simulink model "aconserversimulation"  (R2019b)
settings: Solver=FixedStepAuto  StartTime=0.0  StopTime=30  RelTol=1e-3
undefined symbols (not defined in the file or in its folder): Acid, Lead, sigbuilder_block
libraries: powerlib x39, simulink x14, powerlib_extras x9, electricdrivelib x3, re_lib x1
(part 2 of 2)

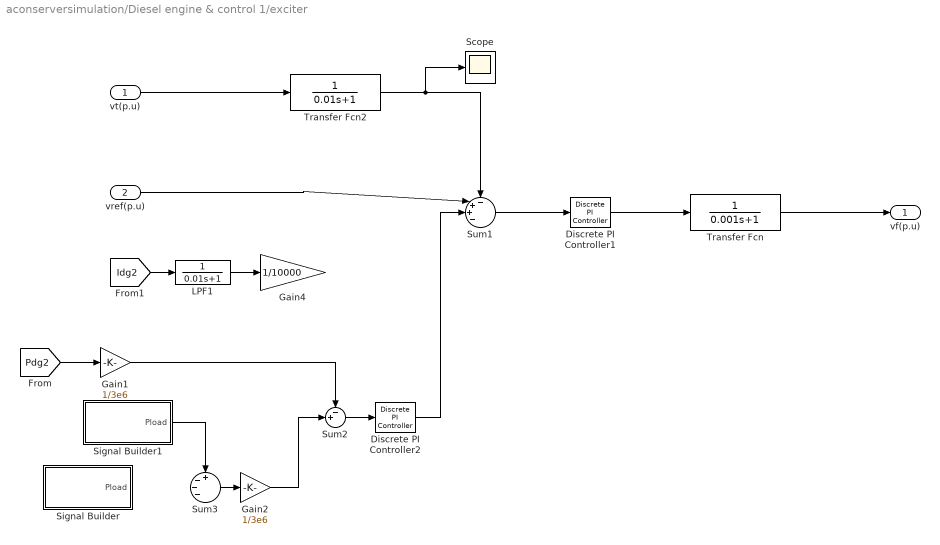
== system aconserversimulation/Diesel engine & control 1/exciter ==
  vt(p.u) : Inport
  vref(p.u) : Inport  Port=2
  Discrete PI Controller1 : powerlib_extras/Discrete  Control Blocks/Discrete PI Controller  Kp=30  Ki=10  Par_Limits=[10 -10]  Init=0  Ts=5e-6
      settings: SourceProductName=Simscape Electrical
  Discrete PI Controller2 : powerlib_extras/Discrete  Control Blocks/Discrete PI Controller  Kp=30  Ki=10  Par_Limits=[10 -10]  Init=0  Ts=5e-6
      settings: SourceProductName=Simscape Electrical
  Gain1 : Gain  Gain=1/3e6
  Gain2 : Gain  Gain=1/3e6
  Gain4 : Gain  Gain=1/10000
  LPF1 : TransferFcn  Denominator=[0.01 1]
  Scope : Scope
  Signal Builder : Subsystem  Tag=STV Subsys  LoadFcn=sigbuilder_block('load');  StartFcn=sigbuilder_block('start');  StopFcn=sigbuilder_block('stop');  ClipboardFcn=sigbuilder_block('clipboard');  mask(Sigbuilder block){tuvar=[0:10]}
      mask help: Simulink:masks:SigbuilderBlock_MD
      mask init:
      | if ~strcmp(get_param(bdroot(gcbh),'SimulationStatus'),'stopped') tuvar = sigbuilder_block('maskInit'); end
      settings: CopyFcn=sigbuilder_block('copy');  DeleteFcn=sigbuilder_block('delete');  ModelCloseFcn=sigbuilder_block('modelClose');  PreSaveFcn=sigbuilder_block('preSave');  PauseFcn=sigbuilder_block('pause');  ContinueFcn=sigbuilder_block('continue');  NameChangeFcn=sigbuilder_block('namechange');  OpenFcn=sigbuilder_block('open',[381.6 135 550.8 400.2 ]);  CloseFcn=sigbuilder_block('close');
      mask Display: plot(0, 0, 100, 100,[2, 2, 32, 32, 2], [68, 8, 8, 68, 68],[32, 2], [38, 38], [32, 19, 2],[53, 60, 44], [32, 17, 17, 2],[16, 16, 31, 31]);txt = getActiveGroup(gcbh);text(2, 100, txt,'verticalAlignment', 'top');
  Signal Builder1 : Subsystem  Tag=STV Subsys  LoadFcn=sigbuilder_block('load');  StartFcn=sigbuilder_block('start');  StopFcn=sigbuilder_block('stop');  ClipboardFcn=sigbuilder_block('clipboard');  mask(Sigbuilder block){tuvar=[0:10]}
      mask help: Simulink:masks:SigbuilderBlock_MD
      mask init:
      | if ~strcmp(get_param(bdroot(gcbh),'SimulationStatus'),'stopped') tuvar = sigbuilder_block('maskInit'); end
      settings: CopyFcn=sigbuilder_block('copy');  DeleteFcn=sigbuilder_block('delete');  ModelCloseFcn=sigbuilder_block('modelClose');  PreSaveFcn=sigbuilder_block('preSave');  PauseFcn=sigbuilder_block('pause');  ContinueFcn=sigbuilder_block('continue');  NameChangeFcn=sigbuilder_block('namechange');  OpenFcn=sigbuilder_block('open',[381.6 135 550.8 400.2 ]);  CloseFcn=sigbuilder_block('close');
      mask Display: plot(0, 0, 100, 100,[2, 2, 32, 32, 2], [68, 8, 8, 68, 68],[32, 2], [38, 38], [32, 19, 2],[53, 60, 44], [32, 17, 17, 2],[16, 16, 31, 31]);txt = getActiveGroup(gcbh);text(2, 100, txt,'verticalAlignment', 'top');
  Sum1 : Sum  Inputs=-++-|
  Sum2 : Sum  Inputs=-+|
  Sum3 : Sum  Inputs=+---|
  Transfer Fcn : TransferFcn  Denominator=[0.001 1]
  Transfer Fcn2 : TransferFcn  Denominator=[0.01 1]
  vf(p.u) : Outport  VectorParamsAs1DForOutWhenUnconnected=off
  wires:
  vt(p.u)/1 -> Transfer Fcn2/1
  Sum1/1 -> Discrete PI Controller1/1
  Discrete PI Controller1/1 -> Transfer Fcn/1
  Transfer Fcn/1 -> vf(p.u)/1
  vref(p.u)/1 -> Sum1/2
  Transfer Fcn2/1 -> Scope/1, Sum1/1
  Sum2/1 -> Discrete PI Controller2/1
  [Pdg2] -> Gain1/1
  Gain1/1 -> Sum2/1
  [Idg2] -> LPF1/1
  LPF1/1 -> Gain4/1
  Discrete PI Controller2/1 -> Sum1/3
  Sum3/1 -> Gain2/1
  Gain2/1 -> Sum2/2
  Signal Builder1/1(Pload) -> Sum3/1

== system aconserversimulation/SC2/Buck-Boost 1  ==
  Vbus_ref : Inport
  Vbus_mes : Inport  Port=2
  Buck-Boost : Subsystem
  Current Measurement : powerlib/Measurements/Current Measurement  PhasorSimulation=off  OutputType=Complex  PSBequivalent=0
      settings: SourceProductName=Simscape Electrical
  Current loop : Subsystem
  Scope3 : Scope
  Voltage loop : Subsystem
  Vout+ : PMIOPort  Side=Right
  Vin+ : PMIOPort  Port=2  Side=Left
  Vout- : PMIOPort  Port=3  Side=Right
  Vin- : PMIOPort  Port=4  Side=Left
  wires:
  Current Measurement/1 -> Current loop/2(iLmes)
  Vbus_mes/1 -> Voltage loop/2(Vmes)
  Vbus_ref/1 -> Voltage loop/1(Vref)
  Current loop/1(d) -> Buck-Boost/1(d)
  Voltage loop/1(iLref) -> Scope3/1, Current loop/1(iLref)
  connections:
  Buck-Boost/RConn1 -- Vout+/RConn1
  Buck-Boost/RConn2 -- Vout-/RConn1
  Vin-/RConn1 -- Buck-Boost/LConn2
  Current Measurement/RConn1 -- Buck-Boost/LConn1
  Current Measurement/LConn1 -- Vin+/RConn1

== system aconserversimulation/Subsystem/Signal Builder ==
  Demux : Demux  Tag=STV Demux  Outputs=1
  FromWs : FromWorkspace  Tag=STV FromWs  VariableName=tuvar  SampleTime=0
      SigBuilderData=|
      | common.afterFinalStr = 'Extrapolate'
      | common.sampleTime = 0
      | dataSet.timeRange = [0 30]
      | dataSet.name = 'Group 1'
      | sbobj.Groups.Name = 'Group 1'
      | sbobj.Groups.Signals.Name = 'Pload'
      | sbobj.Groups.Signals.XData = [0 10 14 16 18.75 21 21 26 26 30]
      | sbobj.Groups.Signals.YData = [0 0 3000000 3000000 6000000 6000000 2000000 2000000 6000000 6020000]
      | sbobj.Groups.TimeRange = [0 30]
  Pload : Outport  Tag=STV Outport  VectorParamsAs1DForOutWhenUnconnected=off
  wires:
  Demux/1 -> Pload/1
  FromWs/1 -> Demux/1

== system aconserversimulation/Battery_V/Buck-Boost 2/Buck-Boost ==
  d : Inport
  Add2 : Sum  Inputs=+-
  Constant : Constant
  Mosfet1 : powerlib/Power Electronics/Mosfet  Ron=0.1  Lon=0  Rd=0.01  Vfd=0  IC=0  Rs=1e5  Cs=inf  Measurements=on
      settings: SourceProductName=Simscape Electrical
  Mosfet3 : powerlib/Power Electronics/Mosfet  Ron=0.1  Lon=0  Rd=0.01  Vfd=0  IC=0  Rs=1e5  Cs=inf  Measurements=on
      settings: SourceProductName=Simscape Electrical
  Relational Operator : RelationalOperator  OutDataTypeStr=boolean  RndMeth=Nearest
  Repeating Sequence : simulink/Sources/Repeating Sequence  rep_seq_t=[0 0.0005 0.001]  rep_seq_y=[0 1 0]
  Terminator : Terminator
  Terminator1 : Terminator
  Vout+ : PMIOPort  Side=Right
  Vout- : PMIOPort  Port=2  Side=Right
  Vin+ : PMIOPort  Port=3  Side=Left
  Vin- : PMIOPort  Port=4  Side=Left
  wires:
  Relational Operator/1 -> Mosfet1/1, Add2/2
  Repeating Sequence/1 -> Relational Operator/2
  Constant/1 -> Add2/1
  Add2/1 -> Mosfet3/1
  Mosfet1/1 -> Terminator1/1
  Mosfet3/1 -> Terminator/1
  d/1 -> Relational Operator/1
  connections:
  Mosfet1/RConn1 -- Vin-/RConn1 -- Vout-/RConn1
  Mosfet3/RConn1 -- Vin+/RConn1 -- Mosfet1/LConn1
  Vout+/RConn1 -- Mosfet3/LConn1

== system aconserversimulation/Battery_V/Buck-Boost 2/Current loop ==
  note: 原p/i=0.0015/0.2
  Iref : Inport
  imes : Inport  Port=2
  Add1 : Sum  Inputs=+-
  Discrete PID Controller1 : simulink/Continuous/PID Controller  Controller=PI  Form=Parallel  TimeDomain=Continuous-time  SampleTime=-1  IntegratorMethod=Forward Euler  FilterMethod=Forward Euler  ControllerParametersSource=internal  P=1.5  I=1  D=0  UseFilter=on  N=100  TunerSelectOption=Transfer Function Based (PID Tuner App)  InitialConditionSource=internal  InitialConditionForIntegrator=0  InitialConditionForFilter=0  DifferentiatorICPrevScaledInput=0  ExternalReset=none  TrackingMode=off  Kt=1  LimitOutput=off  UpperSaturationLimit=inf  LowerSaturationLimit=-inf  LinearizeAsGain=off  AntiWindupMode=none  Kb=1  POutMin=[]  POutMax=[]  IOutMin=[]  IOutMax=[]  DOutMin=[]  DOutMax=[]  NOutMin=[]  NOutMax=[]  SumOutMin=[]  SumOutMax=[]  SaturationOutMin=[]  SaturationOutMax=[]  PParamMin=[]  PParamMax=[]  IParamMin=[]  IParamMax=[]  DParamMin=[]  DParamMax=[]  NParamMin=[]  NParamMax=[]  KbParamMin=[]  KbParamMax=[]  KtParamMin=[]  KtParamMax=[]  KbOutMin=[]  KbOutMax=[]  KtOutMin=[]  KtOutMax=[]  IntegratorOutMin=[]  IntegratorOutMax=[]  FilterOutMin=[]  FilterOutMax=[]  SumI1OutMin=[]  SumI1OutMax=[]  SumI2OutMin=[]  SumI2OutMax=[]  SumI3OutMin=[]  SumI3OutMax=[]  SumI4OutMin=[]  SumI4OutMax=[]  SumDOutMin=[]  SumDOutMax=[]  DifferentiatorOutMin=[]  DifferentiatorOutMax=[]  FilterDiffOutCoefMin=[]  FilterDiffOutCoefMax=[]  ReciprocalOutMin=[]  ReciprocalOutMax=[]  SumDenOutMin=[]  SumDenOutMax=[]  SumNumOutMin=[]  SumNumOutMax=[]  DivideOutMin=[]  DivideOutMax=[]  IntegratorContinuousStateAttributes=''  IntegratorStateMustResolveToSignalObject=off  IntegratorRTWStateStorageClass=Auto  FilterContinuousStateAttributes=''  FilterStateMustResolveToSignalObject=off  FilterRTWStateStorageClass=Auto  ParallelPVariant=InternalParameters  IdealPVariant=Disabled  IVariant=InternalParameters  DVariant=Disabled  IntegratorVariant=Continuous  SatVariant=Disabled  AWVariant=Passthrough  PCopyVariant=Disabled  TRVariant=Disabled  FdbkBlocksVariant=Forward  IdealPFdbkVariant=Disabled  SatFdbkVariant=Disabled  DerivativeFilterVariant=Disabled  NVariant=Disabled  NCopyVariant=Disabled_SignalSpec  FilterICVariant=Disabled  IntegratorICVariant=InternalICs  ExternalResetVariant=Disabled  TRSumVariant=Passthrough  SumFdbkVariant=Disabled  SumVariant=Sum_PI
  d : Outport  VectorParamsAs1DForOutWhenUnconnected=off
  wires:
  Discrete PID Controller1/1 -> d/1
  imes/1 -> Add1/2
  Add1/1 -> Discrete PID Controller1/1
  Iref/1 -> Add1/1

== system aconserversimulation/Battery_V/Buck-Boost 2/Current loop1 ==
  note: 原p/i=0.0015/0.2
  Iref : Inport
  imes : Inport  Port=2
  Add1 : Sum  Inputs=+-
  Discrete PID Controller1 : simulink/Continuous/PID Controller  Controller=PI  TimeDomain=Continuous-time  SampleTime=-1  IntegratorMethod=Forward Euler  FilterMethod=Forward Euler  Form=Parallel  UseFilter=on  ControllerParametersSource=internal  P=100  I=10  D=0  N=100  InitialConditionSource=internal  InitialConditionForIntegrator=0  InitialConditionForFilter=0  ExternalReset=none  LimitOutput=off  UpperSaturationLimit=inf  LowerSaturationLimit=-inf  LinearizeAsGain=off  AntiWindupMode=none  Kb=1  TrackingMode=off  Kt=1  PParamMin=[]  PParamMax=[]  IParamMin=[]  IParamMax=[]  DParamMin=[]  DParamMax=[]  NParamMin=[]  NParamMax=[]  KbParamMin=[]  KbParamMax=[]  KtParamMin=[]  KtParamMax=[]  POutMin=[]  POutMax=[]  IOutMin=[]  IOutMax=[]  DOutMin=[]  DOutMax=[]  NOutMin=[]  NOutMax=[]  KbOutMin=[]  KbOutMax=[]  KtOutMin=[]  KtOutMax=[]  IntegratorOutMin=[]  IntegratorOutMax=[]  FilterOutMin=[]  FilterOutMax=[]  SumOutMin=[]  SumOutMax=[]  SumI1OutMin=[]  SumI1OutMax=[]  SumI2OutMin=[]  SumI2OutMax=[]  SumI3OutMin=[]  SumI3OutMax=[]  SumDOutMin=[]  SumDOutMax=[]  SaturationOutMin=[]  SaturationOutMax=[]  IntegratorContinuousStateAttributes=''  IntegratorStateMustResolveToSignalObject=off  IntegratorRTWStateStorageClass=Auto  FilterContinuousStateAttributes=''  FilterStateMustResolveToSignalObject=off  FilterRTWStateStorageClass=Auto  DifferentiatorICPrevScaledInput=0  DifferentiatorOutMin=[]  DifferentiatorOutMax=[]  InitialConditionSetting=State (most efficient)  FilterDiffOutCoefMin=[]  FilterDiffOutCoefMax=[]  SumDenOutMin=[]  SumDenOutMax=[]  SumNumOutMin=[]  SumNumOutMax=[]  ReciprocalOutMin=[]  ReciprocalOutMax=[]  DivideOutMin=[]  DivideOutMax=[]  TunerSelectOption=Transfer Function Based (PID Tuner App)
  Saturation : Saturate  UpperLimit=500  LowerLimit=-500
  Scope : Scope
  d : Outport  VectorParamsAs1DForOutWhenUnconnected=off
  wires:
  Discrete PID Controller1/1 -> Saturation/1
  imes/1 -> Add1/2
  Add1/1 -> Discrete PID Controller1/1
  Iref/1 -> Add1/1
  [P] -> Scope/1
  Saturation/1 -> d/1

== system aconserversimulation/Battery_V/Buck-Boost 2/Voltage loop ==
  Vref : Inport
  Vmes : Inport  Port=2
  Add : Sum  Inputs=+-
  Discrete PI Controller : powerlib_extras/Discrete  Control Blocks/Discrete PI Controller  Kp=10  Ki=10  Par_Limits=[500 -500]  Init=0  Ts=5e-6
      settings: SourceProductName=Simscape Electrical
  Discrete PID Controller1 : simulink/Continuous/PID Controller  Controller=PI  Form=Parallel  TimeDomain=Continuous-time  SampleTime=-1  IntegratorMethod=Forward Euler  FilterMethod=Forward Euler  ControllerParametersSource=internal  P=10  I=10  D=0  UseFilter=on  N=100  TunerSelectOption=Transfer Function Based (PID Tuner App)  InitialConditionSource=internal  InitialConditionForIntegrator=0  InitialConditionForFilter=0  DifferentiatorICPrevScaledInput=0  ExternalReset=none  TrackingMode=off  Kt=1  LimitOutput=off  UpperSaturationLimit=inf  LowerSaturationLimit=-inf  LinearizeAsGain=off  AntiWindupMode=none  Kb=1  POutMin=[]  POutMax=[]  IOutMin=[]  IOutMax=[]  DOutMin=[]  DOutMax=[]  NOutMin=[]  NOutMax=[]  SumOutMin=[]  SumOutMax=[]  SaturationOutMin=[]  SaturationOutMax=[]  PParamMin=[]  PParamMax=[]  IParamMin=[]  IParamMax=[]  DParamMin=[]  DParamMax=[]  NParamMin=[]  NParamMax=[]  KbParamMin=[]  KbParamMax=[]  KtParamMin=[]  KtParamMax=[]  KbOutMin=[]  KbOutMax=[]  KtOutMin=[]  KtOutMax=[]  IntegratorOutMin=[]  IntegratorOutMax=[]  FilterOutMin=[]  FilterOutMax=[]  SumI1OutMin=[]  SumI1OutMax=[]  SumI2OutMin=[]  SumI2OutMax=[]  SumI3OutMin=[]  SumI3OutMax=[]  SumI4OutMin=[]  SumI4OutMax=[]  SumDOutMin=[]  SumDOutMax=[]  DifferentiatorOutMin=[]  DifferentiatorOutMax=[]  FilterDiffOutCoefMin=[]  FilterDiffOutCoefMax=[]  ReciprocalOutMin=[]  ReciprocalOutMax=[]  SumDenOutMin=[]  SumDenOutMax=[]  SumNumOutMin=[]  SumNumOutMax=[]  DivideOutMin=[]  DivideOutMax=[]  IntegratorContinuousStateAttributes=''  IntegratorStateMustResolveToSignalObject=off  IntegratorRTWStateStorageClass=Auto  FilterContinuousStateAttributes=''  FilterStateMustResolveToSignalObject=off  FilterRTWStateStorageClass=Auto  ParallelPVariant=InternalParameters  IdealPVariant=Disabled  IVariant=InternalParameters  DVariant=Disabled  IntegratorVariant=Continuous  SatVariant=Disabled  AWVariant=Passthrough  PCopyVariant=Disabled  TRVariant=Disabled  FdbkBlocksVariant=Forward  IdealPFdbkVariant=Disabled  SatFdbkVariant=Disabled  DerivativeFilterVariant=Disabled  NVariant=Disabled  NCopyVariant=Disabled_SignalSpec  FilterICVariant=Disabled  IntegratorICVariant=InternalICs  ExternalResetVariant=Disabled  TRSumVariant=Passthrough  SumFdbkVariant=Disabled  SumVariant=Sum_PI
  HPF2 : TransferFcn  Denominator=[2 1]
  Iref : Outport  VectorParamsAs1DForOutWhenUnconnected=off
  wires:
  Vref/1 -> Add/1
  Vmes/1 -> Add/2
  Discrete PI Controller/1 -> Iref/1
  Add/1 -> HPF2/1
  HPF2/1 -> Discrete PI Controller/1

== system aconserversimulation/Diesel engine & control /exciter/Signal Builder ==
  Demux : Demux  Tag=STV Demux  Outputs=1
  FromWs : FromWorkspace  Tag=STV FromWs  VariableName=tuvar  SampleTime=0
      SigBuilderData=|
      | common.afterFinalStr = 'Extrapolate'
      | common.sampleTime = 0
      | dataSet.timeRange = [0 20]
      | dataSet.name = 'Group 1'
      | sbobj.Groups.Name = 'Group 1'
      | sbobj.Groups.Signals.Name = 'Pload'
      | sbobj.Groups.Signals.XData = [0 4 6 6.45 12 12 16 16 20]
      | sbobj.Groups.Signals.YData = [0.195 3000000 3000000 3000000 3000000 1500000 1500000 3000000 3000000]
      | sbobj.Groups.TimeRange = [0 20]
  Pload : Outport  Tag=STV Outport  VectorParamsAs1DForOutWhenUnconnected=off
  wires:
  Demux/1 -> Pload/1
  FromWs/1 -> Demux/1

== system aconserversimulation/Diesel engine & control /exciter/Signal Builder1 ==
  Demux : Demux  Tag=STV Demux  Outputs=1
  FromWs : FromWorkspace  Tag=STV FromWs  VariableName=tuvar  SampleTime=0
      SigBuilderData=|
      | common.afterFinalStr = 'Extrapolate'
      | common.sampleTime = 0
      | dataSet.timeRange = [0 30]
      | dataSet.name = 'Group 1'
      | sbobj.Groups.Name = 'Group 1'
      | sbobj.Groups.Signals.Name = 'Pload'
      | sbobj.Groups.Signals.XData = [0 10 14 16 16.45 22 22 26 26 30]
      | sbobj.Groups.Signals.YData = [0 0 2500000 2500000 3000000 3000000 1500000 1500000 3000000 3000000]
      | sbobj.Groups.TimeRange = [0 30]
  Pload : Outport  Tag=STV Outport  VectorParamsAs1DForOutWhenUnconnected=off
  wires:
  Demux/1 -> Pload/1
  FromWs/1 -> Demux/1

== system aconserversimulation/Diesel engine & control 1/exciter/Signal Builder ==
  Demux : Demux  Tag=STV Demux  Outputs=1
  FromWs : FromWorkspace  Tag=STV FromWs  VariableName=tuvar  SampleTime=0
      SigBuilderData=|
      | common.afterFinalStr = 'Extrapolate'
      | common.sampleTime = 0
      | dataSet.timeRange = [0 20]
      | dataSet.name = 'Group 1'
      | sbobj.Groups.Name = 'Group 1'
      | sbobj.Groups.Signals.Name = 'Pload'
      | sbobj.Groups.Signals.XData = [0 4 6 8.75 12 12 16 16 20]
      | sbobj.Groups.Signals.YData = [0.195 0 0 2500000 2500000 0 0 2500000 2500000]
      | sbobj.Groups.TimeRange = [0 20]
  Pload : Outport  Tag=STV Outport  VectorParamsAs1DForOutWhenUnconnected=off
  wires:
  Demux/1 -> Pload/1
  FromWs/1 -> Demux/1

== system aconserversimulation/Diesel engine & control 1/exciter/Signal Builder1 ==
  Demux : Demux  Tag=STV Demux  Outputs=1
  FromWs : FromWorkspace  Tag=STV FromWs  VariableName=tuvar  SampleTime=0
      SigBuilderData=|
      | common.afterFinalStr = 'Extrapolate'
      | common.sampleTime = 0
      | dataSet.timeRange = [0 30]
      | dataSet.name = 'Group 1'
      | sbobj.Groups.Name = 'Group 1'
      | sbobj.Groups.Signals.Name = 'Pload'
      | sbobj.Groups.Signals.XData = [0 4 16 18.75 22 22 26 26 30]
      | sbobj.Groups.Signals.YData = [0.195 0 0 2500000 2500000 0 0 2500000 2500000]
      | sbobj.Groups.TimeRange = [0 30]
  Pload : Outport  Tag=STV Outport  VectorParamsAs1DForOutWhenUnconnected=off
  wires:
  Demux/1 -> Pload/1
  FromWs/1 -> Demux/1

== system aconserversimulation/SC2/Buck-Boost 1 /Buck-Boost ==
  note: d
  note: 1-d
  d : Inport
  Constant : Constant
  L : powerlib/Elements/Series RLC Branch  LConnTagsString=__new0  RConnTagsString=__new0  BranchType=L  Resistance=1  Inductance=9e-3  SetiL0=off  InitialCurrent=0  Capacitance=1e-6  Setx0=off  InitialVoltage=0  Measurements=Branch current
      settings: SourceProductName=Simscape Electrical
  Mosfet : powerlib/Power Electronics/Mosfet  Ron=0.0001  Lon=0  Rd=0.0001  Vfd=0  IC=0  Rs=1e5  Cs=inf  Measurements=on
      settings: SourceProductName=Simscape Electrical
  Mosfet1 : powerlib/Power Electronics/Mosfet  Ron=0.0001  Lon=0  Rd=0.0001  Vfd=0  IC=0  Rs=1e5  Cs=inf  Measurements=on
      settings: SourceProductName=Simscape Electrical
  Relational Operator1 : RelationalOperator  OutDataTypeStr=boolean  RndMeth=Nearest
  Repeating Sequence1 : simulink/Sources/Repeating Sequence  rep_seq_t=[0 5e-4 1e-3]  rep_seq_y=[0 1 0]
  Sum : Sum  Inputs=|-+
  Vin+ : PMIOPort  Side=Left
  Vin- : PMIOPort  Port=2  Side=Left
  Vout+ : PMIOPort  Port=3  Side=Right
  Vout- : PMIOPort  Port=4  Side=Right
  wires:
  Constant/1 -> Sum/2
  Repeating Sequence1/1 -> Relational Operator1/2
  d/1 -> Relational Operator1/1
  Relational Operator1/1 -> Mosfet/1, Sum/1
  Sum/1 -> Mosfet1/1
  connections:
  Mosfet/RConn1 -- Vout-/RConn1 -- Vin-/RConn1
  Mosfet/LConn1 -- Mosfet1/RConn1 -- L/RConn1
  L/LConn1 -- Vin+/RConn1
  Vout+/RConn1 -- Mosfet1/LConn1

== system aconserversimulation/SC2/Buck-Boost 1 /Current loop ==
  note: 原p/i=0.28/40
  iLref : Inport
  iLmes : Inport  Port=2
  PID Controller : simulink/Continuous/PID Controller  Controller=PI  Form=Ideal  TimeDomain=Continuous-time  SampleTime=-1  IntegratorMethod=Forward Euler  FilterMethod=Forward Euler  ControllerParametersSource=internal  P=0.0045  I=0.20  D=0  UseFilter=on  N=100  TunerSelectOption=Transfer Function Based (PID Tuner App)  InitialConditionSource=internal  InitialConditionForIntegrator=0  InitialConditionForFilter=0  DifferentiatorICPrevScaledInput=0  ExternalReset=none  TrackingMode=off  Kt=1  LimitOutput=off  UpperSaturationLimit=inf  LowerSaturationLimit=-inf  LinearizeAsGain=on  AntiWindupMode=none  Kb=1  POutMin=[]  POutMax=[]  IOutMin=[]  IOutMax=[]  DOutMin=[]  DOutMax=[]  NOutMin=[]  NOutMax=[]  SumOutMin=[]  SumOutMax=[]  SaturationOutMin=[]  SaturationOutMax=[]  PParamMin=[]  PParamMax=[]  IParamMin=[]  IParamMax=[]  DParamMin=[]  DParamMax=[]  NParamMin=[]  NParamMax=[]  KbParamMin=[]  KbParamMax=[]  KtParamMin=[]  KtParamMax=[]  KbOutMin=[]  KbOutMax=[]  KtOutMin=[]  KtOutMax=[]  IntegratorOutMin=[]  IntegratorOutMax=[]  FilterOutMin=[]  FilterOutMax=[]  SumI1OutMin=[]  SumI1OutMax=[]  SumI2OutMin=[]  SumI2OutMax=[]  SumI3OutMin=[]  SumI3OutMax=[]  SumI4OutMin=[]  SumI4OutMax=[]  SumDOutMin=[]  SumDOutMax=[]  DifferentiatorOutMin=[]  DifferentiatorOutMax=[]  FilterDiffOutCoefMin=[]  FilterDiffOutCoefMax=[]  ReciprocalOutMin=[]  ReciprocalOutMax=[]  SumDenOutMin=[]  SumDenOutMax=[]  SumNumOutMin=[]  SumNumOutMax=[]  DivideOutMin=[]  DivideOutMax=[]  IntegratorContinuousStateAttributes=''  IntegratorStateMustResolveToSignalObject=off  IntegratorRTWStateStorageClass=Auto  FilterContinuousStateAttributes=''  FilterStateMustResolveToSignalObject=off  FilterRTWStateStorageClass=Auto  ParallelPVariant=Passthrough  IdealPVariant=InternalParameters  IVariant=InternalParameters  DVariant=Disabled  IntegratorVariant=Continuous  SatVariant=Disabled  AWVariant=Passthrough  PCopyVariant=Disabled  TRVariant=Disabled  FdbkBlocksVariant=Forward  IdealPFdbkVariant=Disabled  SatFdbkVariant=Disabled  DerivativeFilterVariant=Disabled  NVariant=Disabled  NCopyVariant=Disabled_SignalSpec  FilterICVariant=Disabled  IntegratorICVariant=InternalICs  ExternalResetVariant=Disabled  TRSumVariant=Passthrough  SumFdbkVariant=Disabled  SumVariant=Sum_PI
  Subtract : Sum  Inputs=+-
  d : Outport  VectorParamsAs1DForOutWhenUnconnected=off
  wires:
  iLmes/1 -> Subtract/2
  iLref/1 -> Subtract/1
  Subtract/1 -> PID Controller/1
  PID Controller/1 -> d/1

== system aconserversimulation/SC2/Buck-Boost 1 /Voltage loop ==
  note: 原p/i=2.5/40
  Vref : Inport
  Vmes : Inport  Port=2
  HPF2 : TransferFcn  Numerator=[2 0]  Denominator=[2 1]
  PID Controller : simulink/Continuous/PID Controller  Controller=PI  Form=Ideal  TimeDomain=Continuous-time  SampleTime=-1  IntegratorMethod=Forward Euler  FilterMethod=Forward Euler  ControllerParametersSource=internal  P=2  I=1  D=0  UseFilter=on  N=100  TunerSelectOption=Transfer Function Based (PID Tuner App)  InitialConditionSource=internal  InitialConditionForIntegrator=0  InitialConditionForFilter=0  DifferentiatorICPrevScaledInput=0  ExternalReset=none  TrackingMode=off  Kt=1  LimitOutput=off  UpperSaturationLimit=inf  LowerSaturationLimit=-inf  LinearizeAsGain=on  AntiWindupMode=none  Kb=1  POutMin=[]  POutMax=[]  IOutMin=[]  IOutMax=[]  DOutMin=[]  DOutMax=[]  NOutMin=[]  NOutMax=[]  SumOutMin=[]  SumOutMax=[]  SaturationOutMin=[]  SaturationOutMax=[]  PParamMin=[]  PParamMax=[]  IParamMin=[]  IParamMax=[]  DParamMin=[]  DParamMax=[]  NParamMin=[]  NParamMax=[]  KbParamMin=[]  KbParamMax=[]  KtParamMin=[]  KtParamMax=[]  KbOutMin=[]  KbOutMax=[]  KtOutMin=[]  KtOutMax=[]  IntegratorOutMin=[]  IntegratorOutMax=[]  FilterOutMin=[]  FilterOutMax=[]  SumI1OutMin=[]  SumI1OutMax=[]  SumI2OutMin=[]  SumI2OutMax=[]  SumI3OutMin=[]  SumI3OutMax=[]  SumI4OutMin=[]  SumI4OutMax=[]  SumDOutMin=[]  SumDOutMax=[]  DifferentiatorOutMin=[]  DifferentiatorOutMax=[]  FilterDiffOutCoefMin=[]  FilterDiffOutCoefMax=[]  ReciprocalOutMin=[]  ReciprocalOutMax=[]  SumDenOutMin=[]  SumDenOutMax=[]  SumNumOutMin=[]  SumNumOutMax=[]  DivideOutMin=[]  DivideOutMax=[]  IntegratorContinuousStateAttributes=''  IntegratorStateMustResolveToSignalObject=off  IntegratorRTWStateStorageClass=Auto  FilterContinuousStateAttributes=''  FilterStateMustResolveToSignalObject=off  FilterRTWStateStorageClass=Auto  ParallelPVariant=Passthrough  IdealPVariant=InternalParameters  IVariant=InternalParameters  DVariant=Disabled  IntegratorVariant=Continuous  SatVariant=Disabled  AWVariant=Passthrough  PCopyVariant=Disabled  TRVariant=Disabled  FdbkBlocksVariant=Forward  IdealPFdbkVariant=Disabled  SatFdbkVariant=Disabled  DerivativeFilterVariant=Disabled  NVariant=Disabled  NCopyVariant=Disabled_SignalSpec  FilterICVariant=Disabled  IntegratorICVariant=InternalICs  ExternalResetVariant=Disabled  TRSumVariant=Passthrough  SumFdbkVariant=Disabled  SumVariant=Sum_PI
  Subtract : Sum  Inputs=+-
  iLref : Outport  VectorParamsAs1DForOutWhenUnconnected=off
  wires:
  Vmes/1 -> Subtract/2
  Vref/1 -> Subtract/1
  PID Controller/1 -> iLref/1
  Subtract/1 -> HPF2/1
  HPF2/1 -> PID Controller/1
